simulink model "arch2014jin_AbstractFuelControl_M2"  (R2014a)
settings: Solver=ode15s  SolverMode=SingleTasking  StartTime=0.0  StopTime=50  FixedStep=.00005  RelTol=1e-6  AbsTol=1e-6
PreLoadFcn:
  | % model parameters
  |     c1 = 0.41328
  |     c2 = -0.366
  |     c3 = 0.08979
  |     c4 = -0.0337
  |     c5 = 0.0001
  |     c6 = 2.821
  |     c7 = -0.05231
  |     c8 = 0.10299
  |     c9 = -0.00063
  |     c10 = 1.0
  |     c11 = 14.7
  |     c12 = 0.9
  |     c13 = 0.04
  |     c14 = 0.14
  | % coefficients of polynomial approximations
  |     c15 = 13.893
  |     c16 = -35.2518
  |     c17 = 20.7364
  |     c18 = 2.6287
  |     c19 = -1.592
  |     c20 = -2.3421
  |     c21 = 2.7799
  |     c22 = -0.3273
  | % sensors and actuatorerror factor
  |     c23 = 1.0
  |     c24 = 1.0
  |     c25 = 1.0
Description:
  | Modeling Engine Timing Using Triggered Subsystems
  | 
  | This example presents a model of a four-cylinder spark ignition engine
  | and demonstrates Simulink(R) capabilities to model an internal combustion
  | engine from the throttle to the crankshaft output. We used well-defined
  | physical principles supplemented, where appropriate, with empirical
  | relationships that describe the systems dynamic behavior without
  | introducing unnecessary complexity.
settings Model: CovMetricSettings=d  ExtModeTrigMode=oneshot  ExtModeArmWhenConnect=off  ExtModeAutoUpdateStatusClock=off  Creator=The MathWorks Inc.  LastModifiedBy=tjohnson
settings DataIOCC: ExternalInput=[simTime, en_speed]  InitialState=[]  LimitDataPoints=off  SignalLoggingSaveFormat=ModelDataLogs  SaveOutput=off  SignalLogging=off  SaveTime=off  StateSaveName=x  TimeSaveName=t  OutputSaveName=y  SignalLoggingName=sldemo_engine_output
settings OptimizationCC: BlockReduction=off  BooleanDataType=off  ExpressionDepthLimit=2147483647  InitFltsAndDblsToZero=on  BufferReusableBoundary=off
settings DebuggingCC: SignalInfNanChecking=warning  AlgebraicLoopMsg=none  SaveWithParameterizedLinksMsg=none  UnderspecifiedInitializationDetection=Classic  SignalResolutionControl=TryResolveAllWithWarning  SolverPrmCheckMsg=none  InheritedTsInSrcMsg=none  MultiTaskDSMMsg=warning  MultiTaskCondExecSysMsg=none  SigSpecEnsureSampleTimeMsg=none  IntegerOverflowMsg=none  ParameterPrecisionLossMsg=none  FcnCallInpInsideContextMsg=UseLocalSettings  UniqueDataStoreMsg=warning  StateNameClashWarn=warning
settings RTWCC: IncludeERTFirstTime=on
settings GRTTargetCC: TargetFcnLib=ansi_tfl_tmw.mat  CombineOutputUpdateFcns=off  GRTInterface=on

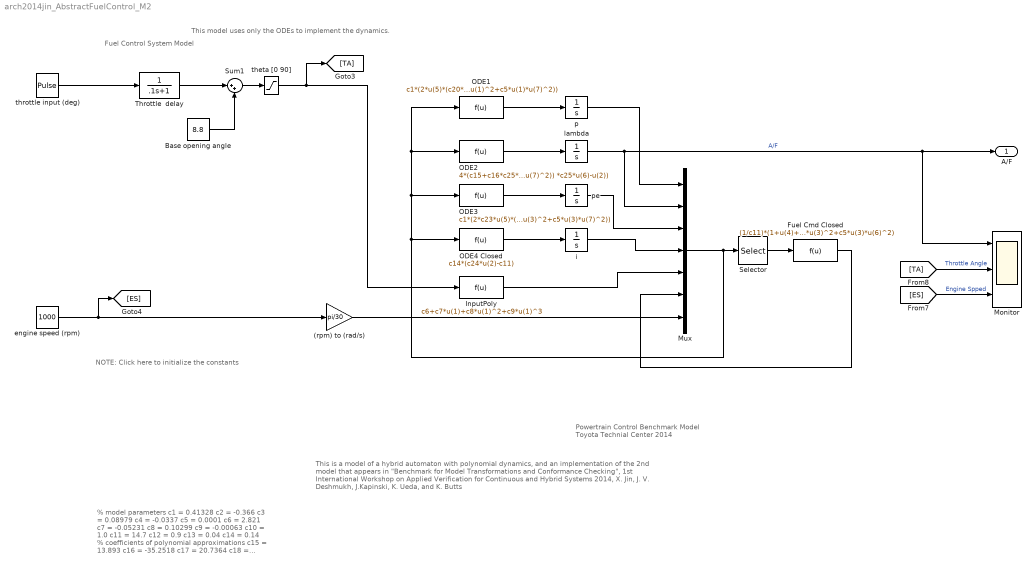
== system arch2014jin_AbstractFuelControl_M2 ==
  note: % model parameters
      |     c1 = 0.41328
      |     c2 = -0.366
      |     c3 = 0.08979
      |     c4 = -0.0337
      |     c5 = 0.0001
      |     c6 = 2.821
      |     c7 = -0.05231
      |     c8 = 0.10299
      |     c9 = -0.00063
      |     c10 = 1.0
      |     c11 = 14.7
      |     c12 = 0.9
      |     c13 = 0.04
      |     c14 = 0.14
      | % coefficients of polynomial approximations
      |     c15 = 13.893
      |     c16 = -35.2518
      |     c17 = 20.7364
      |     c18 = 2.6287
      |     c19 = -1.592
      |     c20 = -2.3421
      |     c21 = 2.7799
      |     c22 = -0.3273
      | % sensors and actuatorerror factor
      |     c23 = 1.0
      |     c24 = 1.0
      |     c25 = 1.0
  note: This model uses only the ODEs to implement the dynamics.
  note: Fuel Control System Model
  note: This is a model of a hybrid automaton with polynomial dynamics, and an implementation of the 2nd model that appears in
      | "Benchmark for Model Transformations and Conformance Checking", 1st International Workshop on Applied Verification for Continuous and Hybrid Systems 2014,
      | X. Jin, J. V. Deshmukh, J.Kapinski, K. Ueda, and K. Butts
  note: Powertrain Control Benchmark Model
      | Toyota Technial Center
      | 2014
  note: NOTE: Click here to initialize the constants
  (rpm) to (rad/s) : Gain  Gain=pi/30
  Base opening angle : Constant  Value=8.8
  Fuel Cmd Closed : Fcn  Expr=(1/c11)*(1+u(4)+c13*(c24*u(2)-c11))*(c2+c3*u(6)*u(3)+c4*u(6)*u(3)^2+c5*u(3)*u(6)^2)
  InputPoly : Fcn  Expr=c6+c7*u(1)+c8*u(1)^2+c9*u(1)^3
  Monitor : Scope  NumInputPorts=3
      settings: TimeRange=50  YMin=12.5~2850~5  YMax=20.5~3150~90
  Mux : Mux  Inputs=7
  ODE1 : Fcn  Expr=c1*(2*u(5)*(c20*u(1)^2+c21*u(1)+c22) - c12*(c2+c3*u(7)*u(1)+c4*u(7)*u(1)^2+c5*u(1)*u(7)^2))
  ODE2 : Fcn  Expr=4*(c15+c16*c25*u(6)+c17*c25^2*u(6)^2+c18*(c12*(c2+c3*u(7)*u(1)+c4*u(7)*u(1)^2+c5*u(1)*u(7)^2)) +c19*(c12*(c2+c3*u(7)*u(1)+c4*u(7)*u(1)^2+c5*u(1)*u(7)^2)) *c25*u(6)-u(2))
  ODE3 : Fcn  Expr=c1*(2*c23*u(5)*(c20*u(1)^2+c21*u(1)+c22)-(c2+c3*u(7)*u(3)+c4*u(7)*u(3)^2+c5*u(3)*u(7)^2))
  ODE4 Closed : Fcn  Expr=c14*(c24*u(2)-c11)
  Selector : Selector  InputPortWidth=7  Indices=[1 2 3 4 5 7]
  Sum1 : Sum  Inputs=|++
  Throttle  delay : TransferFcn  Denominator=[.1 1]
  engine speed (rpm) : Constant  Description=[1000, 3000]  Value=1000
      settings: AttributesFormatString=%<Description>
  i : Integrator  InitialCondition=0.017
  lambda : Integrator  InitialCondition=14.7
  p : Integrator  InitialCondition=0.6353
  pe : Integrator  InitialCondition=0.5573
  theta [0 90] : Saturate  UpperLimit=90  LowerLimit=0
  throttle input (deg) : DiscretePulseGenerator  Description=[0, 81.2]  PulseType=Time based  Amplitude=75.2996  Period=15.7139  PulseWidth=50  PhaseDelay=3
      settings: AttributesFormatString=%<Description>
  A/F : Outport
  wires:
  ODE1/1 -> p/1
  Mux/1 -> ODE1/1, ODE2/1, ODE3/1, ODE4 Closed/1, Selector/1
  InputPoly/1 -> Mux/5
  ODE2/1 -> lambda/1
  p/1 -> Mux/1
  pe/1 -> Mux/3
  i/1 -> Mux/4
  lambda/1 -> Mux/2, Monitor/1, A/F/1  "A/F"
  Fuel Cmd Closed/1 -> Mux/6
  ODE4 Closed/1 -> i/1
  ODE3/1 -> pe/1
  (rpm) to (rad/s)/1 -> Mux/7
  Base opening angle/1 -> Sum1/2
  throttle input (deg)/1 -> Throttle  delay/1
  Throttle  delay/1 -> Sum1/1
  Sum1/1 -> theta [0 90]/1
  theta [0 90]/1 -> [TA], InputPoly/1
  [TA] -> Monitor/2  "Throttle Angle"
  [ES] -> Monitor/3  "Engine Spped"
  engine speed (rpm)/1 -> [ES], (rpm) to (rad/s)/1
  Selector/1 -> Fuel Cmd Closed/1
